simulink model "ISO"  (R2018b)
settings: Solver=VariableStepAuto  StartTime=0.0  StopTime=10.0  RelTol=1e-3
settings Model: Creator=kekos  LastModifiedBy=kekos

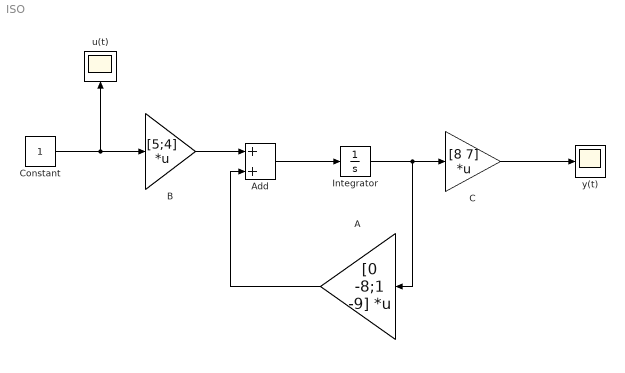
== system ISO ==
  " u(t)" : Scope
  A : Gain  Gain=[0 -8;1 -9]  Multiplication=Matrix(K*u)
  Add : Sum
  B : Gain  Gain=[5;4]  Multiplication=Matrix(K*u)
  "C " : Gain  Gain=[8 7]  Multiplication=Matrix(K*u)
  Constant : Constant
  Integrator : Integrator  InitialCondition=[0.6;0.2]
  y(t) : Scope
  wires:
  Constant/1 -> " u(t)"/1, B/1
  B/1 -> Add/1
  Add/1 -> Integrator/1
  Integrator/1 -> A/1, "C "/1
  A/1 -> Add/2
  "C "/1 -> y(t)/1
